simulink model "Filter_cascade_model"  (R2020b)
settings: Solver=FixedStepAuto  StartTime=0.0  StopTime=10.0  FixedStep=0.2  RelTol=1e-3
settings Model: Creator=153  LastModifiedBy=153
settings DataIOCC: LoadExternalInput=on  SaveFormat=Array  SaveOutput=off  SaveTime=off

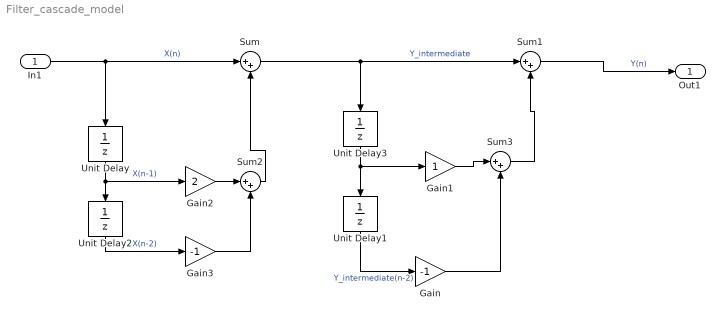
== system Filter_cascade_model ==
  In1 : Inport  OutDataTypeStr=double  PortDimensions=1  SampleTime=[0.20000000000000001,0]
  Gain : Gain  Gain=-1
  Gain1 : Gain
  Gain2 : Gain  Gain=2
  Gain3 : Gain  Gain=-1
  Sum{,1..3} (4 alike) : Sum  Inputs=|++
  Unit Delay{,1..3} (4 alike) : UnitDelay  SampleTime=-1  HasFrameUpgradeWarning=on
  Out1 : Outport  OutDataTypeStr=double  PortDimensions=1  SampleTime=[0.20000000000000001,0]
  wires:
  Unit Delay2/1 -> Gain3/1  "X(n-2)"
  Unit Delay1/1 -> Gain/1  "Y_intermediate(n-2)"
  Gain2/1 -> Sum2/1
  Sum/1 -> Sum1/1, Unit Delay3/1  "Y_intermediate"
  Sum3/1 -> Sum1/2
  Gain/1 -> Sum3/2
  Unit Delay/1 -> Gain2/1, Unit Delay2/1  "X(n-1)"
  Gain1/1 -> Sum3/1
  Unit Delay3/1 -> Unit Delay1/1, Gain1/1
  Gain3/1 -> Sum2/2
  Sum2/1 -> Sum/2
  In1/1 -> Sum/1, Unit Delay/1  "X(n)"
  Sum1/1 -> Out1/1  "Y(n)"
